simulink model "totalSystem_Feedforward"  (R2015b)
settings: Solver=ode45  StartTime=0.0  StopTime=40  RelTol=1e-5
libraries: simulink x1
settings Model: Creator=Labo  LastModifiedBy=thoma
settings DataIOCC: SaveFormat=Array  SignalLoggingSaveFormat=ModelDataLogs  InspectSignalLogs=on
settings DebuggingCC: UnderspecifiedInitializationDetection=Classic  MergeDetectMultiDrivingBlocksExec=none  SolverPrmCheckMsg=warning  MultiTaskDSMMsg=warning  MultiTaskCondExecSysMsg=none  StateNameClashWarn=warning
settings HardwareCC: ProdBitPerPointer=32  ProdLargestAtomicFloat=None  ProdIntDivRoundTo=Undefined  ProdEndianess=Unspecified  ProdWordSize=32  ProdHWDeviceType=32-bit Generic
settings GRTTargetCC: GeneratePreprocessorConditionals=Disable all
settings ConfigComp: CovModelRefEnable=Off

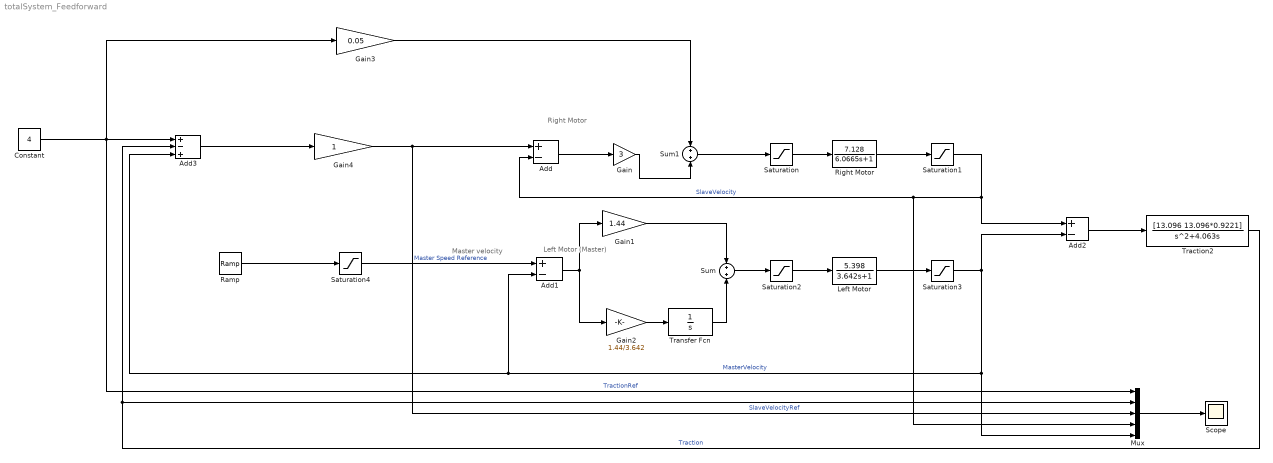
== system totalSystem_Feedforward ==
  note: Master velocity
  note: Left Motor (Master)
  note: Right Motor
  Add : Sum  Inputs=+-
  Add1 : Sum  Inputs=+-
  Add2 : Sum  Inputs=+-
  Add3 : Sum  Inputs=+-+
  Constant : Constant  Value=4
  Gain : Gain  Gain=3
  Gain1 : Gain  Gain=1.44
  Gain2 : Gain  Gain=1.44/3.642
  Gain3 : Gain  Gain=0.05
  Gain4 : Gain
  "Left Motor " : TransferFcn  Numerator=[5.398]  Denominator=[3.642 1]  ContinuousStateAttributes='v'
  Mux : Mux  Inputs=5
  Ramp : simulink/Sources/Ramp  slope=1/16  start=0  X0=0
  "Right Motor " : TransferFcn  Numerator=[7.128]  Denominator=[6.0665 1]  ContinuousStateAttributes='v'
  Saturation : Saturate  UpperLimit=7.3  LowerLimit=-17.3
  Saturation1 : Saturate  UpperLimit=10-2.79  LowerLimit=-10-2.79
  Saturation2 : Saturate  UpperLimit=7.3  LowerLimit=-17.3
  Saturation3 : Saturate  UpperLimit=10-8.623  LowerLimit=-10-8.623
  Saturation4 : Saturate  UpperLimit=2  LowerLimit=0
  "Scope " : Scope
  Sum : Sum  Inputs=+|+
  Sum1 : Sum  Inputs=+|+
  Traction2 : TransferFcn  Numerator=[13.096 13.096*0.9221]  Denominator=[1 4.063 0]
  Transfer Fcn : TransferFcn  Denominator=[1 0]
  wires:
  Add/1 -> Gain/1
  "Right Motor "/1 -> Saturation1/1
  Saturation1/1 -> Add2/1, Mux/4, Add/2  "SlaveVelocity"
  Saturation/1 -> "Right Motor "/1
  Add1/1 -> Gain2/1, Gain1/1
  "Left Motor "/1 -> Saturation3/1
  Saturation3/1 -> Mux/5, Add1/2, Add3/3, Add2/2  "MasterVelocity"
  Saturation2/1 -> "Left Motor "/1
  Sum/1 -> Saturation2/1
  Traction2/1 -> Add3/2, Mux/2  "Traction"
  Constant/1 -> Gain3/1, Add3/1, Mux/1  "TractionRef"
  Saturation4/1 -> Add1/1  "Master Speed Reference"
  Mux/1 -> "Scope "/1
  Add2/1 -> Traction2/1
  Gain2/1 -> Transfer Fcn/1
  Transfer Fcn/1 -> Sum/2
  Gain1/1 -> Sum/1
  Ramp/1 -> Saturation4/1
  Add3/1 -> Gain4/1
  Gain4/1 -> Mux/3, Add/1  "SlaveVelocityRef"
  Gain/1 -> Sum1/2
  Sum1/1 -> Saturation/1
  Gain3/1 -> Sum1/1
